simulink model "power"  (Simulink 7.3)
settings: Solver=ode45  StartTime=0.0  StopTime=10  RelTol=1e-3
undefined symbols (not defined in the file): D1, Delta
libraries: powerlib x22
settings Model: Creator=yadav  LastModifiedBy=yadav

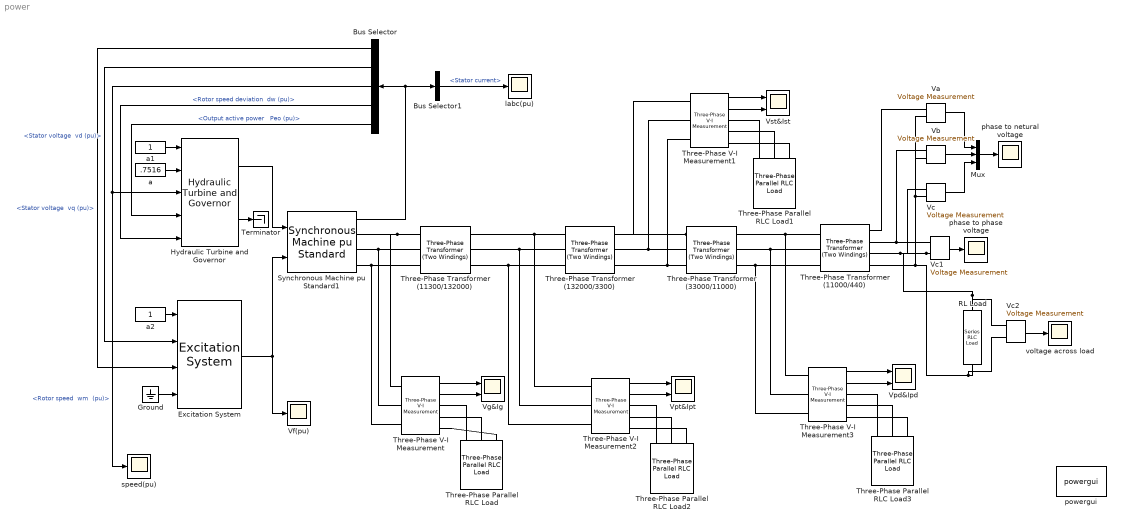
== system power ==
  Bus Selector : BusSelector  OutputSignals="dq0 components.Stator voltage  vq (pu),dq0 components.Stator voltage  vd (pu),Mechanical.Rotor speed  wm  (pu),Mechanical.Rotor speed deviation  dw (pu),Output active power   Peo (pu)"
  Bus Selector1 : BusSelector  OutputSignals=Stator current
  Excitation System : powerlib/Machines/Excitation System  DialogController=POWERSYS.PowerSysDialog  SystemSampleTime=-1  tr=20e-3  reg=[ 300, 0.001 ]  exc=[ 1, 0 ]  tgr=[ 0, 0 ]  damp=[ 0.001, 0.1 ]  sat=[ 0, 0 ]  lim=[ -11.5, 11.5, 0 ]  v0="[1.0  1.28]"
  Ground : Ground
  Hydraulic Turbine and Governor : powerlib/Machines/Hydraulic Turbine and Governor  DialogController=POWERSYS.PowerSysDialog  SystemSampleTime=-1  sm="[ 10/3  0.07 ]"  gate="[  0.01  0.97518  -0.1  0.1 ]"  reg="[  0.05  1.163  0.105  0  0.01  ]"  hyd="[  0  2.67  ]"  dref=0  po=0.7516
  Mux : Mux  Inputs=3
  RL Load : powerlib/Elements/Series RLC Load  DialogController=POWERSYS.PowerSysDialog  PhysicalDomain=powersysdomain  SubClassName=unknown  LeftPortType=p1  RightPortType=p1  LConnTagsString=a  RConnTagsString=__new0  NominalVoltage=1000  NominalFrequency=60  ActivePower=10e3  InductivePower=100  CapacitivePower=0  Setx0=off  InitialVoltage=0  SetiL0=off  InitialCurrent=0  Measurements=None
  Synchronous Machine pu Standard1 : powerlib/Machines/Synchronous Machine pu Standard  DialogController=POWERSYS.PowerSysDialog  SystemSampleTime=-1  PresetModel=No  MechanicalLoad=Mechanical power Pm  ShowDetailedParameters=on  RotorType=Salient-pole  NominalParameters="[ 187E6  13800   50]"  Reactances1=[ 1.81, 0.3, 0.23, 1.76, 0.65, 0.25, 0.15 ]  Reactances2="[ 1.305, 0.296, 0.252, 0.474,  0.243,  0.18 ]"  dAxisTimeConstants=Open-circuit  qAxisTimeConstants=Short-circuit  TimeConstants1="[ 4.4849  0.0681  0.1  ]"  TimeConstants2=[ 8.0, 0.03, 1.0, 0.07 ]  TimeConstants3="[  4.49  0.0681  0.0513  ]"  TimeConstants4=[ 8.0, 0.03, 0.3371, 0.0295 ]  TimeConstants5=[ 1.01, 0.053, 0.1 ]  TimeConstants6=[ 1.3201, 0.023, 1.0, 0.07 ]  TimeConstants7=[0.012 0.003 0.003]  TimeConstants8=[ 1.3201, 0.0231, 0.3371, 0.0295 ]  StatorResistance=0.003  Mechanical="[ 3.7 0  20 ]"  PolePairs=20  InitialConditions="[ 0  0  0  0  0  0  0  0  1 ]"  SetSaturation=off  Saturation=[0.6404,0.7127,0.8441,0.9214,0.9956,1.082,1.19,1.316,1.457;0.7,0.7698,0.8872,0.9466,0.9969,1.046,1.1,1.151,1.201]  Units=per unit standard parameters  LoadFlowParameters=[1,0,0,0,0]  TsPowergui=0  TsBlock=-1  IterativeModel=Forward Euler
  Terminator : Terminator
  Three-Phase Parallel RLC Load{,1..3} (4 alike) : powerlib/Elements/Three-Phase Parallel RLC Load  DialogController=POWERSYS.PowerSysDialog  PhysicalDomain=powersysdomain  SubClassName=unknown  LeftPortType=p1  RightPortType=p1  LConnTagsString=A|B|C  Configuration=Y (grounded)  NominalVoltage=1000  NominalFrequency=60  ActivePower=10e3  InductivePower=100  CapacitivePower=100  Measurements=None
  Three-Phase Transformer (11000/440) : powerlib/Elements/Three-Phase Transformer (Two Windings)  DialogController=POWERSYS.PowerSysDialog  SystemSampleTime=-1  Winding1Connection=Delta (D1)  UNITS=pu  NominalPower=[ 250e6 , 50 ]  Winding1=[ 1100 , 0.002 , 0.08 ]  Winding2Connection=Yn  Winding2=[ 250, 0.002 , 0.08 ]  SetSaturation=off  Rm=500  Lm=500  Saturation=[ 0,0 ; 0.0024,1.2 ; 1.0,1.52 ]  Hysteresis=off  DataFile='hysteresis'  SetInitialFlux=off  InitialFluxes=[ 0.8 , -0.8 , 0.7 ]  Measurements=None  MoreParameters=off  BreakLoop=off  DataType=off  TransfoNumber=1
  Three-Phase Transformer (11300/132000) : powerlib/Elements/Three-Phase Transformer (Two Windings)  DialogController=POWERSYS.PowerSysDialog  SystemSampleTime=-1  Winding1Connection=Delta (D1)  UNITS=pu  NominalPower=[ 187e6 , 50 ]  Winding1=[ 11300 , 0.002 , 0.08 ]  Winding2Connection=Delta (D1)  Winding2=[ 132e3 , 0.002 , 0.08 ]  SetSaturation=off  Rm=500  Lm=500  Saturation=[ 0,0 ; 0.0024,1.2 ; 1.0,1.52 ]  Hysteresis=off  DataFile='hysteresis'  SetInitialFlux=off  InitialFluxes=[ 0.8 , -0.8 , 0.7 ]  Measurements=None  MoreParameters=off  BreakLoop=off  DataType=off  TransfoNumber=1
  Three-Phase Transformer (132000/3300) : powerlib/Elements/Three-Phase Transformer (Two Windings)  DialogController=POWERSYS.PowerSysDialog  SystemSampleTime=-1  Winding1Connection=Delta (D1)  UNITS=pu  NominalPower=[ 187e6 , 50 ]  Winding1=[ 132e3 , 0.002 , 0.08 ]  Winding2Connection=Delta (D1)  Winding2=[ 33000 , 0.002 , 0.08 ]  SetSaturation=off  Rm=500  Lm=500  Saturation=[ 0,0 ; 0.0024,1.2 ; 1.0,1.52 ]  Hysteresis=off  DataFile='hysteresis'  SetInitialFlux=off  InitialFluxes=[ 0.8 , -0.8 , 0.7 ]  Measurements=None  MoreParameters=off  BreakLoop=off  DataType=off  TransfoNumber=1
  Three-Phase Transformer (33000/11000) : powerlib/Elements/Three-Phase Transformer (Two Windings)  DialogController=POWERSYS.PowerSysDialog  SystemSampleTime=-1  Winding1Connection=Delta (D1)  UNITS=pu  NominalPower=[ 187e6 , 50 ]  Winding1=[ 33000 , 0.002 , 0.08 ]  Winding2Connection=Delta (D1)  Winding2=[ 1100 , 0.002 , 0.08 ]  SetSaturation=off  Rm=500  Lm=500  Saturation=[ 0,0 ; 0.0024,1.2 ; 1.0,1.52 ]  Hysteresis=off  DataFile='hysteresis'  SetInitialFlux=off  InitialFluxes=[ 0.8 , -0.8 , 0.7 ]  Measurements=None  MoreParameters=off  BreakLoop=off  DataType=off  TransfoNumber=1
  Three-Phase V-I Measurement{,1..3} (4 alike) : powerlib/Measurements/Three-Phase V-I Measurement  DialogController=POWERSYS.PowerSysDialog  SystemSampleTime=-1  VoltageMeasurement=phase-to-ground  SetLabelV=off  LabelV=Vabc  Vpu=off  CurrentMeasurement=yes  SetLabelI=off  LabelI=Iabc  Ipu=off  Pbase=100e6  Vbase=500e3  OutputType=Complex  PhasorSimulation=off  PSBequivalent=0
  Va : powerlib/Measurements/Voltage Measurement  DialogController=POWERSYS.PowerSysDialog  SystemSampleTime=-1  PhasorSimulation=off  OutputType=Complex  PSBequivalent=0
  Vb : powerlib/Measurements/Voltage Measurement  DialogController=POWERSYS.PowerSysDialog  SystemSampleTime=-1  PhasorSimulation=off  OutputType=Complex  PSBequivalent=0
  Vc : powerlib/Measurements/Voltage Measurement  DialogController=POWERSYS.PowerSysDialog  SystemSampleTime=-1  PhasorSimulation=off  OutputType=Complex  PSBequivalent=0
  Vc1 : powerlib/Measurements/Voltage Measurement  DialogController=POWERSYS.PowerSysDialog  SystemSampleTime=-1  PhasorSimulation=off  OutputType=Complex  PSBequivalent=0
  Vc2 : powerlib/Measurements/Voltage Measurement  DialogController=POWERSYS.PowerSysDialog  SystemSampleTime=-1  PhasorSimulation=off  OutputType=Complex  PSBequivalent=0
  Vf(pu) : Scope
      settings: YMin=4.7  YMax=5.15
  Vg&Ig : Scope  NumInputPorts=2
      settings: TimeRange=0.25  YMin=-12000~-120  YMax=12000~120  SaveName=ScopeData3
  Vpd&Ipd : Scope  NumInputPorts=2
      settings: TimeRange=0.2813875310109952  YMin=-1250~-12.5  YMax=1250~12.5  SaveName=ScopeData8
  Vpt&Ipt : Scope  NumInputPorts=2
      settings: TimeRange=0.2813875310109952  YMin=-150000~-1500  YMax=150000~1500  SaveName=ScopeData5
  Vst&Ist : Scope  NumInputPorts=2
      settings: TimeRange=0.2813875310109952  YMin=-35000~-350  YMax=35000~300  SaveName=ScopeData7
  a : Constant  Value=.7516  OutDataType=fixdt(1, 16)  OutScaling=2^0
  a1 : Constant  OutDataType=fixdt(1, 16)  OutScaling=2^0
  a2 : Constant  OutDataType=fixdt(1, 16)  OutScaling=2^0
  labc(pu) : Scope
      settings: TimeRange=0.1459713444183604  YMin=-1.5  YMax=1.5  SaveName=ScopeData2
  phase to netural voltage : Scope
      settings: TimeRange=0.1683611329198365  YMin=-250  YMax=250  SaveName=ScopeData4
  phase to phase voltage : Scope
      settings: TimeRange=0.1459713444183604  YMin=-450  YMax=450  SaveName=ScopeData6
  powergui : powerlib/powergui  Priority=1  SystemSampleTime=-1  SimulationMode=Continuous  SampleTime=50e-6  frequency=60  SPID=off  DisableSnubberDevices=off  DisableRonSwitches=off  DisableVfSwitches=off  SwTol=0  Interpol=off  frequencyindice=50  echomessages=off  HookPort=off  DisplayEquations=off  FunctionMessages=off  EnableUseOfTLC=off  x0status=blocks  RestoreLinks=warning  Frange=[0:2:500]  Ylog=off  Xlog=on  ShowGrid=off  save=off  variable=ZData  ZoomFFT=on  StartTime=0.0  cycles=1  DisplayStyle=1  fundamental=60  FreqAxis=off  MaxFrequency=1000  frequencyindicesteady=1  RmsSteady=1  display=off  Ts=0  methode=off
  speed(pu) : Scope
      settings: YMin=0.952  YMax=0.965
  voltage across load : Scope
      settings: TimeRange=0.1459713444183604  YMin=-250  YMax=250  SaveName=ScopeData9
  wires:
  Synchronous Machine pu Standard1/1 -> Bus Selector/1, Bus Selector1/1
  Bus Selector/1 -> Excitation System/3  "<Stator voltage  vq (pu)>"
  Bus Selector/2 -> Excitation System/2  "<Stator voltage  vd (pu)>"
  Bus Selector/3 -> Hydraulic Turbine and Governor/3, speed(pu)/1  "<Rotor speed  wm  (pu)>"
  Bus Selector/4 -> Hydraulic Turbine and Governor/5  "<Rotor speed deviation  dw (pu)>"
  Bus Selector/5 -> Hydraulic Turbine and Governor/4  "<Output active power   Peo (pu)>"
  Hydraulic Turbine and Governor/1 -> Synchronous Machine pu Standard1/1
  a1/1 -> Hydraulic Turbine and Governor/1
  a/1 -> Hydraulic Turbine and Governor/2
  a2/1 -> Excitation System/1
  Ground/1 -> Excitation System/4
  Hydraulic Turbine and Governor/2 -> Terminator/1
  Excitation System/1 -> Vf(pu)/1, Synchronous Machine pu Standard1/2
  Bus Selector1/1 -> labc(pu)/1  "<Stator current>"
  Three-Phase V-I Measurement/1 -> Vg&Ig/1
  Three-Phase V-I Measurement/2 -> Vg&Ig/2
  Three-Phase V-I Measurement2/1 -> Vpt&Ipt/1
  Three-Phase V-I Measurement2/2 -> Vpt&Ipt/2
  Vc1/1 -> phase to phase voltage/1
  Three-Phase V-I Measurement1/1 -> Vst&Ist/1
  Three-Phase V-I Measurement1/2 -> Vst&Ist/2
  Three-Phase V-I Measurement3/1 -> Vpd&Ipd/1
  Three-Phase V-I Measurement3/2 -> Vpd&Ipd/2
  Va/1 -> Mux/1
  Vb/1 -> Mux/2
  Vc/1 -> Mux/3
  Mux/1 -> phase to netural voltage/1
  Vc2/1 -> voltage across load/1
  connections:
  Synchronous Machine pu Standard1/RConn1 -- Three-Phase Transformer (11300/132000)/LConn1 -- Three-Phase V-I Measurement/LConn1
  Three-Phase Parallel RLC Load/LConn1 -- Three-Phase V-I Measurement/RConn1
  Three-Phase V-I Measurement/RConn2 -- Three-Phase Parallel RLC Load/LConn2
  Three-Phase V-I Measurement/RConn3 -- Three-Phase Parallel RLC Load/LConn3
  Three-Phase V-I Measurement2/RConn1 -- Three-Phase Parallel RLC Load2/LConn1
  Three-Phase V-I Measurement2/RConn2 -- Three-Phase Parallel RLC Load2/LConn2
  Three-Phase V-I Measurement2/RConn3 -- Three-Phase Parallel RLC Load2/LConn3
  Three-Phase Transformer (11300/132000)/LConn2 -- Synchronous Machine pu Standard1/RConn2 -- Three-Phase V-I Measurement/LConn2
  Synchronous Machine pu Standard1/RConn3 -- Three-Phase Transformer (11300/132000)/LConn3 -- Three-Phase V-I Measurement/LConn3
  Three-Phase Transformer (132000/3300)/RConn1 -- Three-Phase Transformer (33000/11000)/LConn1 -- Three-Phase V-I Measurement1/LConn1
  Three-Phase Transformer (132000/3300)/RConn2 -- Three-Phase Transformer (33000/11000)/LConn2 -- Three-Phase V-I Measurement1/LConn2
  Three-Phase Transformer (132000/3300)/RConn3 -- Three-Phase Transformer (33000/11000)/LConn3 -- Three-Phase V-I Measurement1/LConn3
  Three-Phase Transformer (33000/11000)/RConn1 -- Three-Phase Transformer (11000/440)/LConn1 -- Three-Phase V-I Measurement3/LConn1
  Three-Phase Transformer (33000/11000)/RConn2 -- Three-Phase Transformer (11000/440)/LConn2 -- Three-Phase V-I Measurement3/LConn2
  Three-Phase Transformer (33000/11000)/RConn3 -- Three-Phase Transformer (11000/440)/LConn3 -- Three-Phase V-I Measurement3/LConn3
  Three-Phase V-I Measurement2/LConn1 -- Three-Phase Transformer (132000/3300)/LConn1 -- Three-Phase Transformer (11300/132000)/RConn1
  Three-Phase V-I Measurement2/LConn2 -- Three-Phase Transformer (11300/132000)/RConn2 -- Three-Phase Transformer (132000/3300)/LConn2
  Three-Phase V-I Measurement2/LConn3 -- Three-Phase Transformer (11300/132000)/RConn3 -- Three-Phase Transformer (132000/3300)/LConn3
  Three-Phase Transformer (11000/440)/RConn1 -- Va/LConn1
  Three-Phase Transformer (11000/440)/RConn2 -- Vb/LConn1 -- Vc1/LConn1
  Three-Phase Transformer (11000/440)/RConn3 -- Vc/LConn1 -- Vc1/LConn2 -- RL Load/LConn1 -- Vc2/LConn1
  RL Load/RConn1 -- Three-Phase Transformer (11000/440)/RConn4 -- Va/LConn2 -- Vb/LConn2 -- Vc/LConn2 -- Vc2/LConn2
  Three-Phase V-I Measurement1/RConn2 -- Three-Phase Parallel RLC Load1/LConn2
  Three-Phase V-I Measurement1/RConn1 -- Three-Phase Parallel RLC Load1/LConn1
  Three-Phase V-I Measurement1/RConn3 -- Three-Phase Parallel RLC Load1/LConn3
  Three-Phase V-I Measurement3/RConn2 -- Three-Phase Parallel RLC Load3/LConn2
  Three-Phase V-I Measurement3/RConn1 -- Three-Phase Parallel RLC Load3/LConn1
  Three-Phase V-I Measurement3/RConn3 -- Three-Phase Parallel RLC Load3/LConn3
